simulink model "Q4_30"  (R2015b)
settings: Solver=VariableStepAuto  StartTime=0.0  StopTime=5.0  RelTol=1e-3
settings Model: Creator=sam  LastModifiedBy=sam

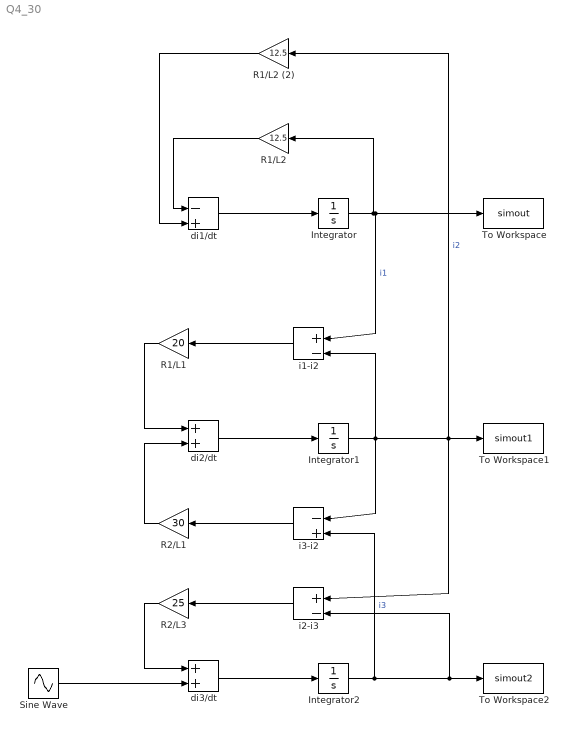
== system Q4_30 ==
  Integrator : Integrator
  Integrator1 : Integrator
  Integrator2 : Integrator
  R1/L1 : Gain  Gain=20
  R1/L2 : Gain  Gain=12.5
  R1/L2 (2) : Gain  Gain=12.5
  R2/L1 : Gain  Gain=30
  R2/L3 : Gain  Gain=25
  Sine Wave : Sin  Amplitude=3.33333  Frequency=6  SampleTime=0
  To Workspace : ToWorkspace  VariableName=simout  SaveFormat=Timeseries  SampleTime=-1
  To Workspace1 : ToWorkspace  VariableName=simout1  SaveFormat=Timeseries  SampleTime=-1
  To Workspace2 : ToWorkspace  VariableName=simout2  SaveFormat=Timeseries  SampleTime=-1
  di1/dt : Sum  Inputs=-|+
  di2/dt : Sum
  di3/dt : Sum
  i1-i2 : Sum  Inputs=+|-
  i2-i3 : Sum  Inputs=+|-
  i3-i2 : Sum  Inputs=-|+
  wires:
  di1/dt/1 -> Integrator/1
  di2/dt/1 -> Integrator1/1
  di3/dt/1 -> Integrator2/1
  Integrator/1 -> R1/L2/1, i1-i2/1, To Workspace/1  "i1"
  Integrator1/1 -> i3-i2/1, i1-i2/2, i2-i3/1, R1/L2 (2)/1, To Workspace1/1  "i2"
  Integrator2/1 -> i3-i2/2, i2-i3/2, To Workspace2/1  "i3"
  R1/L2/1 -> di1/dt/1
  R1/L2 (2)/1 -> di1/dt/2
  i1-i2/1 -> R1/L1/1
  R1/L1/1 -> di2/dt/1
  i3-i2/1 -> R2/L1/1
  R2/L1/1 -> di2/dt/2
  i2-i3/1 -> R2/L3/1
  R2/L3/1 -> di3/dt/1
  Sine Wave/1 -> di3/dt/2
